simulink model "model_electric_damper"  (R2020a)
settings: Solver=ode15s  StartTime=0.0  StopTime=120  MaxStep=0.005  RelTol=1e-3
model workspace (MATLAB code in the model file):
  | eps = 8.854e-12;
  | A = 0.015;
  | Rl = 1;
  | phi1 = 3.63;
  | phi2 = 5.35;
  | e = 1;
settings Model: Creator=Barath Krishna S  LastModifiedBy=dell

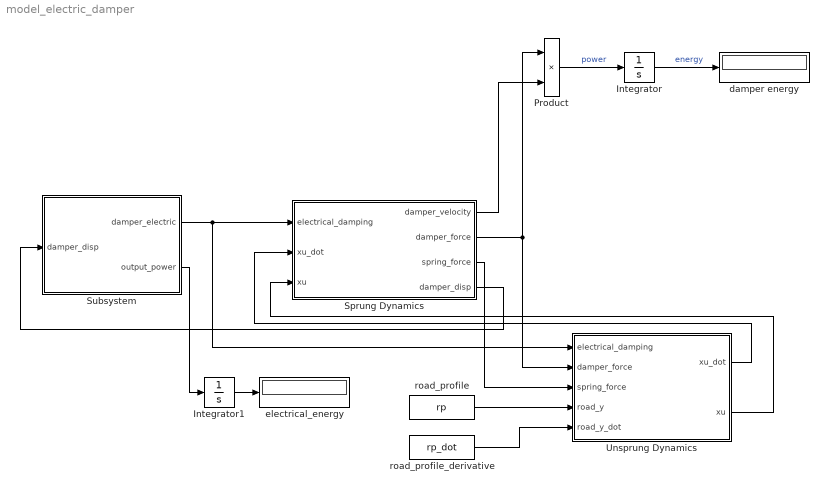
== system model_electric_damper ==
  Integrator : Integrator
  Integrator1 : Integrator
  Product : Product
  Sprung Dynamics : Subsystem
  Subsystem : Subsystem
  Unsprung Dynamics : Subsystem
  damper energy : Display
      settings: Decimation=2
  electrical_energy : Display
      settings: Decimation=2
  road_profile : FromWorkspace  VariableName=rp
  road_profile_derivative : FromWorkspace  VariableName=rp_dot
  wires:
  Product/1 -> Integrator/1  "power"
  Sprung Dynamics/2(damper_force) -> Product/1, Unsprung Dynamics/2(damper_force)
  Sprung Dynamics/1(damper_velocity) -> Product/2
  Sprung Dynamics/3(spring_force) -> Unsprung Dynamics/3(spring_force)
  road_profile/1 -> Unsprung Dynamics/4(road_y)
  road_profile_derivative/1 -> Unsprung Dynamics/5(road_y_dot)
  Unsprung Dynamics/1(xu_dot) -> Sprung Dynamics/2(xu_dot)
  Unsprung Dynamics/2(xu) -> Sprung Dynamics/3(xu)
  Sprung Dynamics/4(damper_disp) -> Subsystem/1(damper_disp)
  Subsystem/1(damper_electric) -> Unsprung Dynamics/1(electrical_damping), Sprung Dynamics/1(electrical_damping)
  Subsystem/2(output_power) -> Integrator1/1
  Integrator/1 -> damper energy/1  "energy"
  Integrator1/1 -> electrical_energy/1

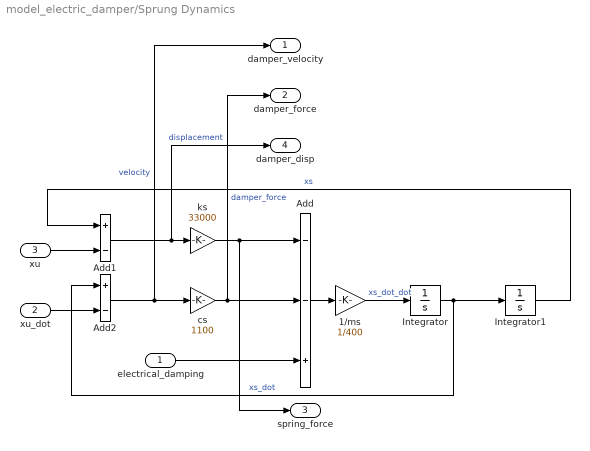
== system model_electric_damper/Sprung Dynamics ==
  electrical_damping : Inport
  xu_dot : Inport  Port=2
  xu : Inport  Port=3
  1/ms : Gain  Gain=1/400
  Add : Sum  Inputs=--+
  Add1 : Sum  Inputs=+-
  Add2 : Sum  Inputs=+-
  Integrator : Integrator
  Integrator1 : Integrator
  cs : Gain  Gain=1100
  ks : Gain  Gain=33000
  damper_velocity : Outport
  damper_force : Outport  Port=2
  spring_force : Outport  Port=3
  damper_disp : Outport  Port=4
  wires:
  1/ms/1 -> Integrator/1  "xs_dot_dot"
  Add2/1 -> damper_velocity/1, cs/1  "velocity"
  ks/1 -> spring_force/1, Add/1
  Add/1 -> 1/ms/1
  Add1/1 -> damper_disp/1, ks/1  "displacement"
  Integrator1/1 -> Add1/1  "xs"
  cs/1 -> Add/2, damper_force/1  "damper_force"
  xu/1 -> Add1/2
  Integrator/1 -> Integrator1/1, Add2/1  "xs_dot"
  xu_dot/1 -> Add2/2
  electrical_damping/1 -> Add/3

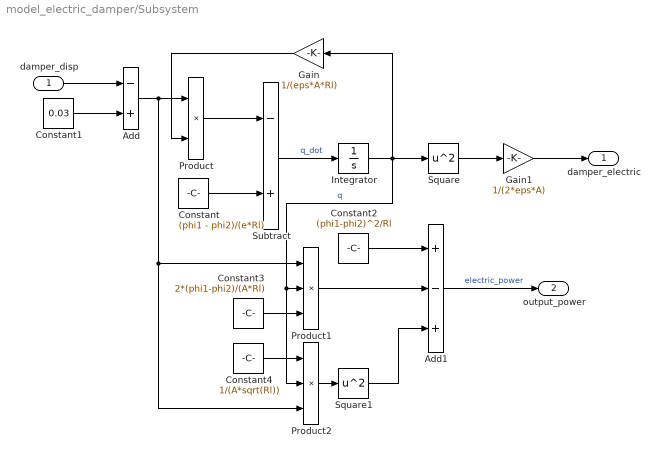
== system model_electric_damper/Subsystem ==
  damper_disp : Inport
  Add : Sum  Inputs=-+
  Add1 : Sum  Inputs=+-+
  Constant : Constant  Value=(phi1 - phi2)/(e*Rl)
  Constant1 : Constant  Value=0.03
  Constant2 : Constant  Value=(phi1-phi2)^2/Rl
  Constant3 : Constant  Value=2*(phi1-phi2)/(A*Rl)
  Constant4 : Constant  Value=1/(A*sqrt(Rl))
  Gain : Gain  Gain=1/(eps*A*Rl)
  Gain1 : Gain  Gain=1/(2*eps*A)
  Integrator : Integrator
  Product : Product
  Product1 : Product  Inputs=3
  Product2 : Product  Inputs=3
  Square : Math  Operator=square  SaturateOnIntegerOverflow=on
  Square1 : Math  Operator=square  SaturateOnIntegerOverflow=on
  Subtract : Sum  Inputs=-+
  damper_electric : Outport
  output_power : Outport  Port=2
  wires:
  Product/1 -> Subtract/1
  Subtract/1 -> Integrator/1  "q_dot"
  Integrator/1 -> Product2/2, Product1/2, Square/1, Gain/1  "q"
  Gain/1 -> Product/2
  Constant/1 -> Subtract/2
  Square/1 -> Gain1/1
  Gain1/1 -> damper_electric/1
  damper_disp/1 -> Add/1
  Constant1/1 -> Add/2
  Constant2/1 -> Add1/1
  Constant3/1 -> Product1/3
  Product1/1 -> Add1/2
  Add/1 -> Product2/3, Product1/1, Product/1
  Constant4/1 -> Product2/1
  Product2/1 -> Square1/1
  Square1/1 -> Add1/3
  Add1/1 -> output_power/1  "electric_power"

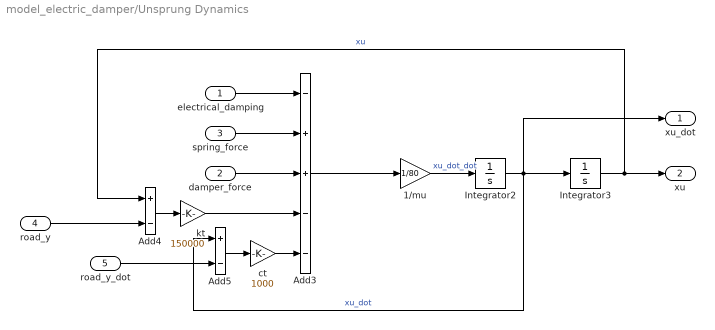
== system model_electric_damper/Unsprung Dynamics ==
  electrical_damping : Inport
  damper_force : Inport  Port=2
  spring_force : Inport  Port=3
  road_y : Inport  Port=4
  road_y_dot : Inport  Port=5
  1/mu : Gain  Gain=1/80
  Add3 : Sum  Inputs=-++--
  Add4 : Sum  Inputs=+-
  Add5 : Sum  Inputs=+-
  Integrator2 : Integrator
  Integrator3 : Integrator
  ct : Gain  Gain=1000
  kt : Gain  Gain=150000
  xu_dot : Outport
  xu : Outport  Port=2
  wires:
  road_y_dot/1 -> Add5/2
  1/mu/1 -> Integrator2/1  "xu_dot_dot"
  kt/1 -> Add3/4
  ct/1 -> Add3/5
  Add3/1 -> 1/mu/1
  Add4/1 -> kt/1
  Add5/1 -> ct/1
  Integrator3/1 -> xu/1, Add4/1  "xu"
  Integrator2/1 -> xu_dot/1, Add5/1, Integrator3/1  "xu_dot"
  damper_force/1 -> Add3/3
  spring_force/1 -> Add3/2
  road_y/1 -> Add4/2
  electrical_damping/1 -> Add3/1
